simulink model "sampleModel16"  (Simulink 9.1)
settings: Solver=VariableStepAuto  StartTime=0.0  StopTime=10.0  RelTol=1e-3
undefined symbols (not defined in the file): DiscIntNeverNeededParam, Newton, Raphson
libraries: simulink x14
settings Model: SuppressorTable="22 serialization::archive 11 0 6 0 0 1 8 0 0 0 0 6 0 0 1 0 21 sampleModel16/cfblk29 0 6 0 0 2 8 0 0 0 0 6 41 Simulink:DataType:WarningOverFlowDetected 0 0 0 6 0  0  0 0 0 0 8 20160608 0 0 0 15 23 17 0 1 40 SimulinkFixedPoint:util:Overflowoccurred 0 0 0  0  8 20160608 0 15 23 17 0 1"  Creator=DELL  LastModifiedBy=DELL
settings DataIOCC: SaveFormat=Dataset
settings OptimizationCC: LifeSpan=auto
settings DebuggingCC: UnderspecifiedInitializationDetection=Simplified  MergeDetectMultiDrivingBlocksExec=error  SFUnexpectedBacktrackingDiag=error  SFNoUnconditionalDefaultTransitionDiag=error  SFExecutionAtInitializationDiag=warning
settings HardwareCC: ProdBitPerPointer=64  ProdBitPerSizeT=64  ProdBitPerPtrDiffT=64  ProdLargestAtomicFloat=Float  ProdIntDivRoundTo=Zero  ProdEndianess=LittleEndian  ProdWordSize=64  ProdHWDeviceType=Intel->x86-64 (Windows64)
settings ModelReferenceCC: PropagateSignalLabelsOutOfModel=on
settings CodeAppCC: StateflowObjectComments=off
settings GRTTargetCC: TargetLangStandard=C99 (ISO)  CombineOutputUpdateFcns=on  GRTInterface=off
settings ConfigComp: CovMetricSettings=dwe  CovHtmlReporting=off  CovSaveCumulativeToWorkspaceVar=off  CovSaveSingleToWorkspaceVar=off  CovExternalEMLEnable=on

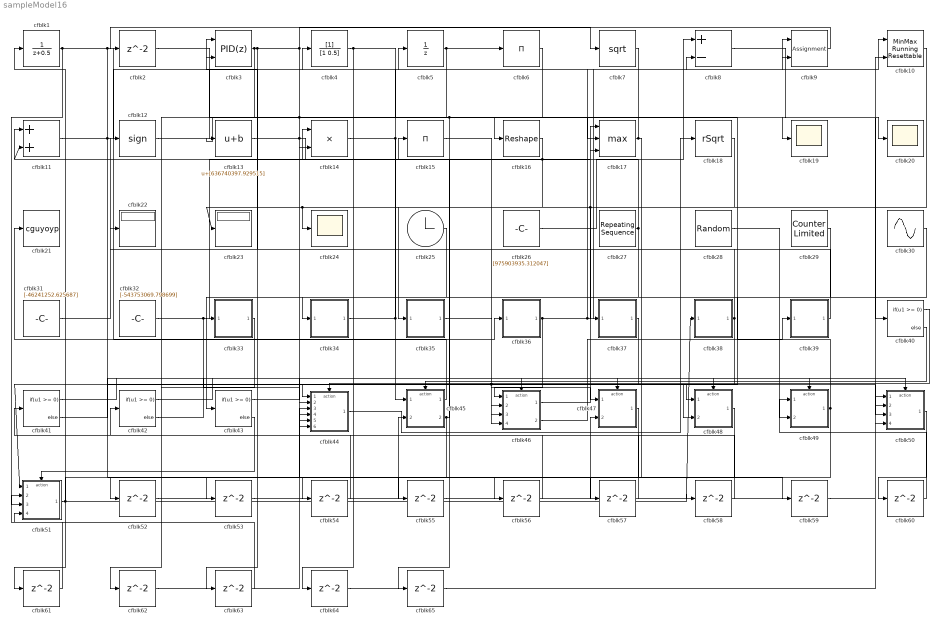
== system sampleModel16 ==
  cfblk1 : DiscreteTransferFcn  SampleTime=1
  cfblk10 : simulink/Math Operations/MinMax Running Resettable  Function=min  vinit=0.0
  cfblk11 : Sum
  cfblk12 : Signum
  cfblk13 : Bias  Bias=[636740397.929515]
  cfblk14 : Product  Inputs=**
  cfblk15 : Product  Inputs=*
  cfblk16 : Reshape
  cfblk17 : MinMax  Function=max  Inputs=3
  cfblk18 : Sqrt  Operator=rSqrt  AlgorithmType=Newton-Raphson  SaturateOnIntegerOverflow=on
  cfblk19 : Scope
  cfblk{2,52..65} (15 alike) : Delay  SampleTime=1
  cfblk20 : Scope
  cfblk21 : ToWorkspace  VariableName=cguyoyp  SaveFormat=Timeseries  SampleTime=-1
  cfblk22 : Display
  cfblk23 : Display
  cfblk24 : Scope
  cfblk25 : Clock
  cfblk26 : Constant  Value=[975903935.312047]  SampleTime=1
  cfblk27 : simulink/Sources/Repeating Sequence  rep_seq_t=[0 2]  rep_seq_y=[-628768262.786288, 33540011.241070]
  cfblk28 : UniformRandomNumber  Minimum=[-3598479047.893037]  Maximum=[8689509005.201536]  Seed=[60011837.000000]  SampleTime=0.1
  cfblk29 : simulink/Sources/Counter Limited  uplimit=[999.000000]  tsamp=-1
  cfblk3 : simulink/Continuous/PID Controller (2DOF)  Controller=PID  TimeDomain=Discrete-time  SampleTime=1  IntegratorMethod=Forward Euler  FilterMethod=Forward Euler  Form=Parallel  UseFilter=on  ControllerParametersSource=internal  P=1  I=1  D=0  N=100  b=1  c=1  InitialConditionSource=internal  InitialConditionForIntegrator=0  InitialConditionForFilter=0  ExternalReset=none  LimitOutput=off  UpperSaturationLimit=inf  LowerSaturationLimit=-inf  LinearizeAsGain=off  AntiWindupMode=none  Kb=1  TrackingMode=off  Kt=1  PParamMin=[]  PParamMax=[]  IParamMin=[]  IParamMax=[]  DParamMin=[]  DParamMax=[]  NParamMin=[]  NParamMax=[]  bParamMin=[]  bParamMax=[]  cParamMin=[]  cParamMax=[]  KbParamMin=[]  KbParamMax=[]  KtParamMin=[]  KtParamMax=[]  POutMin=[]  POutMax=[]  IOutMin=[]  IOutMax=[]  DOutMin=[]  DOutMax=[]  NOutMin=[]  NOutMax=[]  bOutMin=[]  bOutMax=[]  cOutMin=[]  cOutMax=[]  KbOutMin=[]  KbOutMax=[]  KtOutMin=[]  KtOutMax=[]  IntegratorOutMin=[]  IntegratorOutMax=[]  FilterOutMin=[]  FilterOutMax=[]  SumOutMin=[]  SumOutMax=[]  Sum1OutMin=[]  Sum1OutMax=[]  Sum2OutMin=[]  Sum2OutMax=[]  Sum3OutMin=[]  Sum3OutMax=[]  SumI1OutMin=[]  SumI1OutMax=[]  SumI2OutMin=[]  SumI2OutMax=[]  SumI3OutMin=[]  SumI3OutMax=[]  SumDOutMin=[]  SumDOutMax=[]  SaturationOutMin=[]  SaturationOutMax=[]  IntegratorContinuousStateAttributes=''  IntegratorStateMustResolveToSignalObject=off  IntegratorRTWStateStorageClass=Auto  FilterContinuousStateAttributes=''  FilterStateMustResolveToSignalObject=off  FilterRTWStateStorageClass=Auto  DifferentiatorICPrevScaledInput=0  DifferentiatorOutMin=[]  DifferentiatorOutMax=[]  FilterDiffOutCoefMin=[]  FilterDiffOutCoefMax=[]  SumDenOutMin=[]  SumDenOutMax=[]  SumNumOutMin=[]  SumNumOutMax=[]  ReciprocalOutMin=[]  ReciprocalOutMax=[]  DivideOutMin=[]  DivideOutMax=[]  TunerSelectOption=Transfer Function Based (PID Tuner App)
  cfblk30 : Sin  Amplitude=[-741647399.193095]  Bias=[-413258711.550195]  SampleTime=0
  cfblk31 : Constant  Value=[-46241252.625687]  SampleTime=1
  cfblk32 : Constant  Value=[-543753069.798699]  SampleTime=1
  cfblk33 : Subsystem
  cfblk34 : Subsystem
  cfblk35 : Subsystem
  cfblk36 : Subsystem
  cfblk37 : Subsystem
  cfblk38 : Subsystem
  cfblk39 : Subsystem
  cfblk4 : DiscreteFilter  SampleTime=1
  cfblk{40..43} (4 alike) : If  IfExpression=u1 >= 0  SampleTime=1
  cfblk44 : Subsystem  TreatAsAtomicUnit=on
  cfblk45 : Subsystem  TreatAsAtomicUnit=on
  cfblk46 : Subsystem  TreatAsAtomicUnit=on
  cfblk47 : Subsystem  TreatAsAtomicUnit=on
  cfblk48 : Subsystem  TreatAsAtomicUnit=on
  cfblk49 : Subsystem  TreatAsAtomicUnit=on
  cfblk5 : UnitDelay
  cfblk50 : Subsystem  TreatAsAtomicUnit=on
  cfblk51 : Subsystem  TreatAsAtomicUnit=on
  cfblk6 : Product  Inputs=*
  cfblk7 : Sqrt  SaturateOnIntegerOverflow=on
  cfblk8 : Sum  Inputs=+-
  cfblk9 : Assignment  DiagnosticForDimensions=Warning  IndexOptions=Index vector (dialog)  Indices=1  OutputSizes=1
  wires:
  cfblk12/1 -> cfblk5/1
  cfblk32/1 -> cfblk15/1, cfblk44/6(cfblk17)
  cfblk51/1(cfblk2) -> cfblk38/1(cfblk1), cfblk11/1
  cfblk37/1(cfblk2) -> cfblk51/1(cfblk1), cfblk46/2(cfblk10)
  cfblk49/1(cfblk2) -> cfblk13/1, cfblk61/1
  cfblk8/1 -> cfblk20/1
  cfblk1/1 -> cfblk36/1(cfblk1), cfblk50/3(cfblk15), cfblk51/3(cfblk13)
  cfblk9/1 -> cfblk2/1
  cfblk36/1(cfblk2) -> cfblk10/1, cfblk9/1, cfblk46/1(cfblk1)
  cfblk45/1(cfblk2) -> cfblk21/1
  cfblk44/1(cfblk2) -> cfblk18/1
  cfblk29/1 -> cfblk43/1
  cfblk26/1 -> cfblk8/1
  cfblk16/1 -> cfblk23/1, cfblk24/1, cfblk11/2
  cfblk11/1 -> cfblk4/1, cfblk55/1
  cfblk17/1 -> cfblk16/1, cfblk57/1
  cfblk14/1 -> cfblk8/2, cfblk46/3(cfblk11)
  cfblk45/2(cfblk12) -> cfblk14/1, cfblk64/1
  cfblk46/1(cfblk2) -> cfblk17/1
  cfblk38/1(cfblk2) -> cfblk12/1, cfblk44/1(cfblk1)
  cfblk2/1 -> cfblk40/1
  cfblk3/1 -> cfblk7/1, cfblk58/1, cfblk63/1, cfblk62/1
  cfblk31/1 -> cfblk22/1
  cfblk10/1 -> cfblk37/1(cfblk1), cfblk46/4(cfblk12)
  cfblk15/1 -> cfblk47/1(cfblk1)
  cfblk13/1 -> cfblk17/3, cfblk59/1
  cfblk25/1 -> cfblk34/1(cfblk1)
  cfblk5/1 -> cfblk6/1, cfblk14/2
  cfblk27/1 -> cfblk3/1, cfblk44/2(cfblk13)
  cfblk30/1 -> cfblk48/1(cfblk1)
  cfblk7/1 -> cfblk17/2
  cfblk18/1 -> cfblk35/1(cfblk1)
  cfblk28/1 -> cfblk49/2(cfblk17)
  cfblk35/1(cfblk2) -> cfblk48/2(cfblk10)
  cfblk34/1(cfblk2) -> cfblk45/1(cfblk1), cfblk9/2
  cfblk4/1 -> cfblk19/1, cfblk54/1
  cfblk6/1 -> cfblk33/1(cfblk1), cfblk44/4(cfblk15), cfblk65/1
  cfblk46/2(cfblk13) -> cfblk39/1(cfblk1)
  cfblk39/1(cfblk2) -> cfblk3/2
  cfblk40/1 -> cfblk44/Action
  cfblk40/2 -> cfblk45/Action
  cfblk41/1 -> cfblk46/Action
  cfblk41/2 -> cfblk47/Action
  cfblk42/1 -> cfblk48/Action
  cfblk42/2 -> cfblk49/Action
  cfblk43/1 -> cfblk50/Action
  cfblk43/2 -> cfblk51/Action
  cfblk33/1(cfblk2) -> cfblk52/1
  cfblk52/1 -> cfblk10/2
  cfblk48/1(cfblk2) -> cfblk53/1
  cfblk53/1 -> cfblk45/2(cfblk11)
  cfblk54/1 -> cfblk1/1
  cfblk55/1 -> cfblk47/2(cfblk10)
  cfblk47/1(cfblk2) -> cfblk56/1
  cfblk56/1 -> cfblk41/1
  cfblk57/1 -> cfblk44/5(cfblk16)
  cfblk58/1 -> cfblk42/1
  cfblk59/1 -> cfblk50/1(cfblk1)
  cfblk50/1(cfblk2) -> cfblk60/1
  cfblk60/1 -> cfblk49/1(cfblk1)
  cfblk61/1 -> cfblk51/2(cfblk12)
  cfblk62/1 -> cfblk44/3(cfblk14)
  cfblk63/1 -> cfblk51/4(cfblk14)
  cfblk64/1 -> cfblk50/2(cfblk14)
  cfblk65/1 -> cfblk50/4(cfblk16)

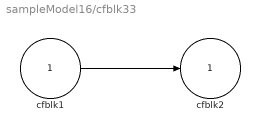
== system sampleModel16/cfblk33 ==
  cfblk1 : Inport
  cfblk2 : Outport
  wires:
  cfblk1/1 -> cfblk2/1

== system sampleModel16/cfblk34 ==
  cfblk1 : Inport
  cfblk2 : Outport
  wires:
  cfblk1/1 -> cfblk2/1

== system sampleModel16/cfblk35 ==
  cfblk1 : Inport
  cfblk2 : Outport
  wires:
  cfblk1/1 -> cfblk2/1

== system sampleModel16/cfblk36 ==
  cfblk1 : Inport
  cfblk2 : Outport
  wires:
  cfblk1/1 -> cfblk2/1

== system sampleModel16/cfblk37 ==
  cfblk1 : Inport
  cfblk2 : Outport
  wires:
  cfblk1/1 -> cfblk2/1

== system sampleModel16/cfblk38 ==
  cfblk1 : Inport
  cfblk2 : Outport
  wires:
  cfblk1/1 -> cfblk2/1

== system sampleModel16/cfblk39 ==
  cfblk1 : Inport
  cfblk2 : Outport
  wires:
  cfblk1/1 -> cfblk2/1

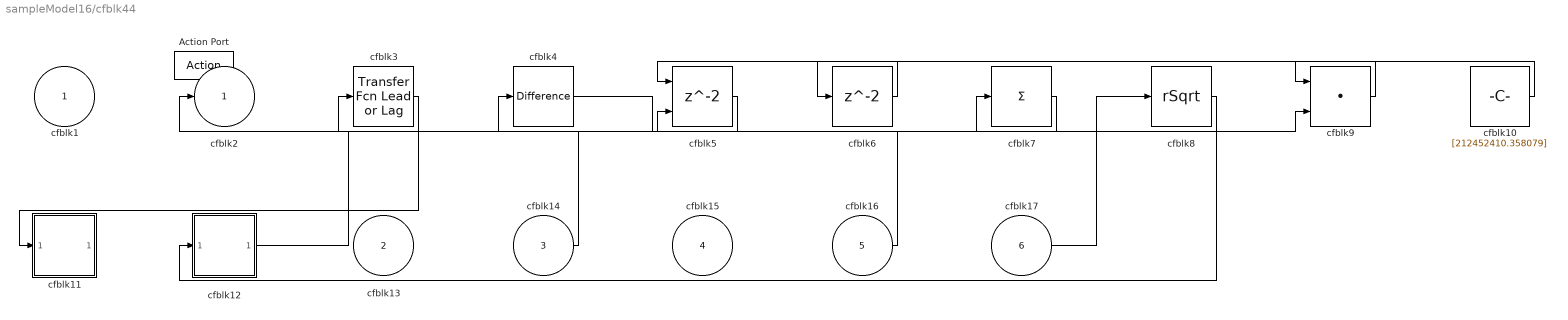
== system sampleModel16/cfblk44 ==
  cfblk1 : Inport
  cfblk13 : Inport  Port=2
  cfblk14 : Inport  Port=3
  cfblk15 : Inport  Port=4
  cfblk16 : Inport  Port=5
  cfblk17 : Inport  Port=6
  Action Port : ActionPort  ActionType=then
  cfblk10 : Constant  Value=[212452410.358079]  SampleTime=1
  cfblk11 : Subsystem
  cfblk12 : Subsystem
  cfblk3 : simulink/Discrete/Transfer Fcn Lead or Lag  PoleZ=0.95  ZeroZ=0.75  ICPrevOutput=0.0  ICPrevInput=0.0  DoSatur=off
      settings: SourceProductName=Simulink  SourceProductBaseCode=SL
  cfblk4 : simulink/Discrete/Difference  ICPrevInput=0.0  OutMin=[]  OutMax=[]  OutDataTypeStr=Inherit: Inherit via back propagation  OutDataType=fixdt(1, 16)  OutScaling=2^-10  DoSatur=off
  cfblk5 : Delay  ShowEnablePort=on
      settings: InputPortMap=u0,e6
  cfblk6 : Delay
  cfblk7 : Sum  Inputs=+
  cfblk8 : Sqrt  Operator=rSqrt  AlgorithmType=Newton-Raphson  SaturateOnIntegerOverflow=on
  cfblk9 : DotProduct  InputSameDT=on  OutDataTypeStr=Inherit: Inherit via internal rule
  cfblk2 : Outport
  wires:
  cfblk3/1 -> cfblk11/1(cfblk1)
  cfblk6/1 -> cfblk5/1
  cfblk14/1 -> cfblk4/1
  cfblk7/1 -> cfblk5/2
  cfblk5/1 -> cfblk2/1
  cfblk10/1 -> cfblk9/1
  cfblk17/1 -> cfblk8/1
  cfblk12/1(cfblk2) -> cfblk7/1
  cfblk8/1 -> cfblk12/1(cfblk1)
  cfblk9/1 -> cfblk6/1
  cfblk4/1 -> cfblk9/2
  cfblk16/1 -> cfblk3/1

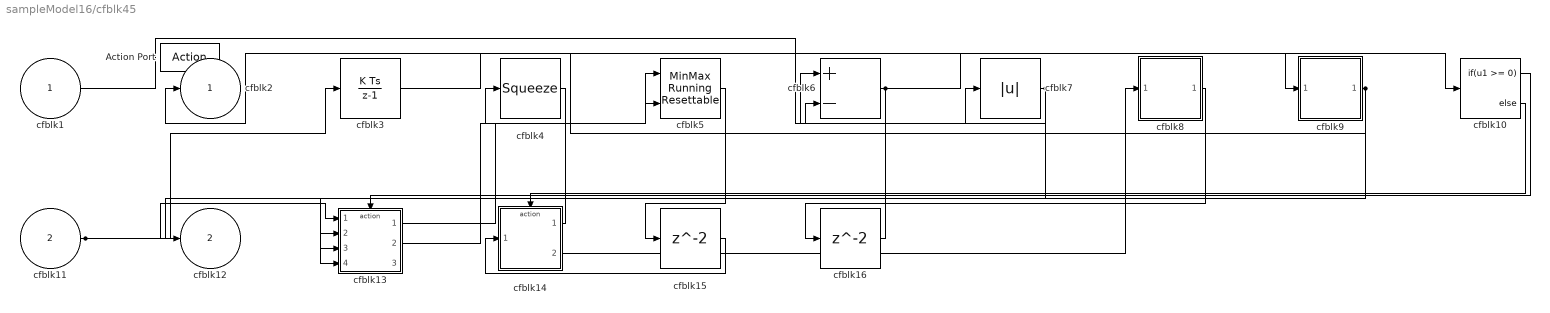
== system sampleModel16/cfblk45 ==
  cfblk1 : Inport
  cfblk11 : Inport  Port=2
  Action Port : ActionPort  ActionType=else
  cfblk10 : If  IfExpression=u1 >= 0  SampleTime=1
  cfblk13 : Subsystem  TreatAsAtomicUnit=on
  cfblk14 : Subsystem  TreatAsAtomicUnit=on
  cfblk15 : Delay
  cfblk16 : Delay
  cfblk3 : DiscreteIntegrator  SampleTime=-1  ICPrevOutput=DiscIntNeverNeededParam  ICPrevScaledInput=DiscIntNeverNeededParam
  cfblk4 : Squeeze
  cfblk5 : simulink/Math Operations/MinMax Running Resettable  Function=min  vinit=0.0
  cfblk6 : Sum  Inputs=+-
  cfblk7 : Abs
  cfblk8 : Subsystem
  cfblk9 : Subsystem
  cfblk2 : Outport
  cfblk12 : Outport  Port=2
  wires:
  cfblk14/1(cfblk2) -> cfblk4/1
  cfblk1/1 -> cfblk7/1
  cfblk9/1(cfblk2) -> cfblk2/1, cfblk13/3(cfblk12)
  cfblk6/1 -> cfblk10/1, cfblk13/2(cfblk11)
  cfblk11/1 -> cfblk3/1, cfblk13/1(cfblk1)
  cfblk14/2(cfblk16) -> cfblk8/1(cfblk1)
  cfblk7/1 -> cfblk6/2, cfblk13/4(cfblk13)
  cfblk4/1 -> cfblk12/1
  cfblk3/1 -> cfblk9/1(cfblk1)
  cfblk13/1(cfblk2) -> cfblk5/1
  cfblk13/2(cfblk14) -> cfblk5/2
  cfblk10/1 -> cfblk13/Action
  cfblk10/2 -> cfblk14/Action
  cfblk5/1 -> cfblk15/1
  cfblk15/1 -> cfblk14/1(cfblk1)
  cfblk8/1(cfblk2) -> cfblk16/1
  cfblk16/1 -> cfblk6/1

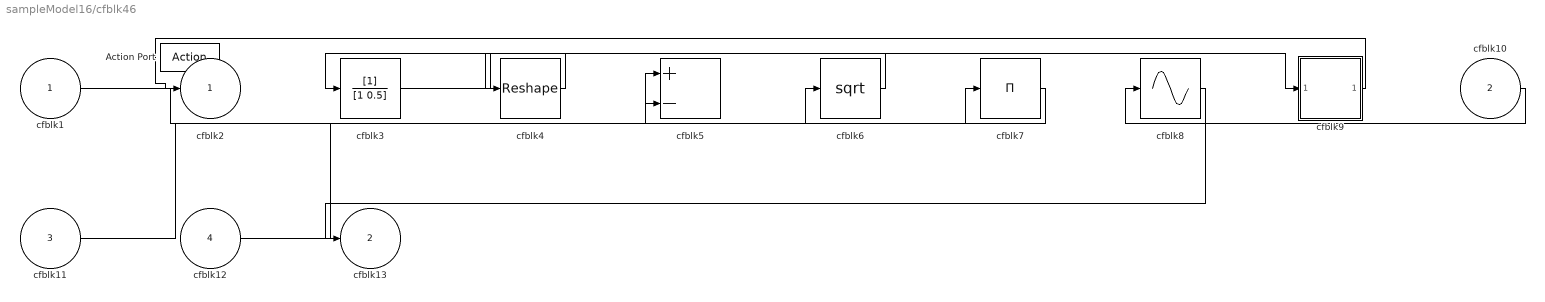
== system sampleModel16/cfblk46 ==
  cfblk1 : Inport
  cfblk10 : Inport  Port=2
  cfblk11 : Inport  Port=3
  cfblk12 : Inport  Port=4
  Action Port : ActionPort  ActionType=then
  cfblk3 : DiscreteFilter
  cfblk4 : Reshape
  cfblk5 : Sum  Inputs=+-
  cfblk6 : Sqrt  SaturateOnIntegerOverflow=on
  cfblk7 : Product  Inputs=*
  cfblk8 : Sin  TimeSource=Use external signal  SampleTime=0
  cfblk9 : Subsystem
  cfblk2 : Outport
  cfblk13 : Outport  Port=2
  wires:
  cfblk12/1 -> cfblk6/1
  cfblk3/1 -> cfblk9/1(cfblk1)
  cfblk4/1 -> cfblk3/1
  cfblk1/1 -> cfblk7/1
  cfblk11/1 -> cfblk5/1
  cfblk10/1 -> cfblk8/1
  cfblk6/1 -> cfblk4/1
  cfblk9/1(cfblk2) -> cfblk2/1
  cfblk8/1 -> cfblk13/1
  cfblk7/1 -> cfblk5/2

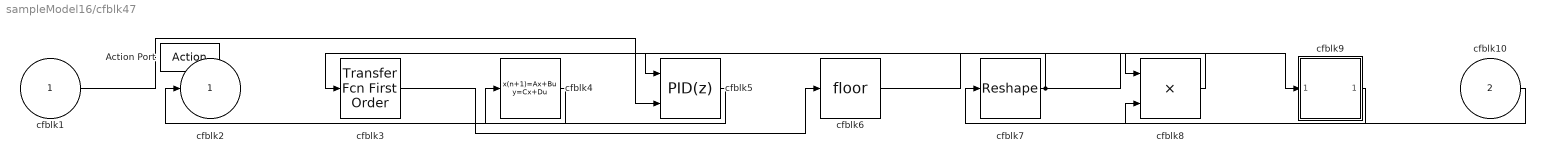
== system sampleModel16/cfblk47 ==
  cfblk1 : Inport
  cfblk10 : Inport  Port=2
  Action Port : ActionPort  ActionType=else
  cfblk3 : simulink/Discrete/Transfer Fcn First Order  PoleZ=0.95  ICPrevOutput=0.0  DoSatur=off
      settings: SourceProductName=Simulink
  cfblk4 : DiscreteStateSpace  SampleTime=-1
  cfblk5 : simulink/Continuous/PID Controller (2DOF)  Controller=PID  TimeDomain=Discrete-time  SampleTime=-1  IntegratorMethod=Forward Euler  FilterMethod=Forward Euler  Form=Parallel  UseFilter=on  ControllerParametersSource=internal  P=1  I=1  D=0  N=100  b=1  c=1  InitialConditionSource=internal  InitialConditionForIntegrator=0  InitialConditionForFilter=0  ExternalReset=none  LimitOutput=off  UpperSaturationLimit=inf  LowerSaturationLimit=-inf  LinearizeAsGain=off  AntiWindupMode=none  Kb=1  TrackingMode=off  Kt=1  PParamMin=[]  PParamMax=[]  IParamMin=[]  IParamMax=[]  DParamMin=[]  DParamMax=[]  NParamMin=[]  NParamMax=[]  bParamMin=[]  bParamMax=[]  cParamMin=[]  cParamMax=[]  KbParamMin=[]  KbParamMax=[]  KtParamMin=[]  KtParamMax=[]  POutMin=[]  POutMax=[]  IOutMin=[]  IOutMax=[]  DOutMin=[]  DOutMax=[]  NOutMin=[]  NOutMax=[]  bOutMin=[]  bOutMax=[]  cOutMin=[]  cOutMax=[]  KbOutMin=[]  KbOutMax=[]  KtOutMin=[]  KtOutMax=[]  IntegratorOutMin=[]  IntegratorOutMax=[]  FilterOutMin=[]  FilterOutMax=[]  SumOutMin=[]  SumOutMax=[]  Sum1OutMin=[]  Sum1OutMax=[]  Sum2OutMin=[]  Sum2OutMax=[]  Sum3OutMin=[]  Sum3OutMax=[]  SumI1OutMin=[]  SumI1OutMax=[]  SumI2OutMin=[]  SumI2OutMax=[]  SumI3OutMin=[]  SumI3OutMax=[]  SumDOutMin=[]  SumDOutMax=[]  SaturationOutMin=[]  SaturationOutMax=[]  IntegratorContinuousStateAttributes=''  IntegratorStateMustResolveToSignalObject=off  IntegratorRTWStateStorageClass=Auto  FilterContinuousStateAttributes=''  FilterStateMustResolveToSignalObject=off  FilterRTWStateStorageClass=Auto  DifferentiatorICPrevScaledInput=0  DifferentiatorOutMin=[]  DifferentiatorOutMax=[]  FilterDiffOutCoefMin=[]  FilterDiffOutCoefMax=[]  SumDenOutMin=[]  SumDenOutMax=[]  SumNumOutMin=[]  SumNumOutMax=[]  ReciprocalOutMin=[]  ReciprocalOutMax=[]  DivideOutMin=[]  DivideOutMax=[]  TunerSelectOption=Transfer Function Based (PID Tuner App)
  cfblk6 : Rounding
  cfblk7 : Reshape
  cfblk8 : Product
  cfblk9 : Subsystem
  cfblk2 : Outport
  wires:
  cfblk8/1 -> cfblk5/1
  cfblk10/1 -> cfblk7/1
  cfblk5/1 -> cfblk4/1
  cfblk1/1 -> cfblk5/2
  cfblk6/1 -> cfblk8/1
  cfblk7/1 -> cfblk3/1, cfblk9/1(cfblk1)
  cfblk3/1 -> cfblk6/1
  cfblk4/1 -> cfblk2/1
  cfblk9/1(cfblk2) -> cfblk8/2

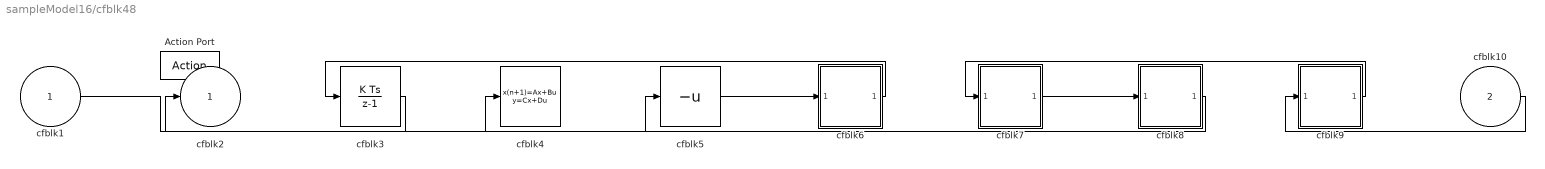
== system sampleModel16/cfblk48 ==
  cfblk1 : Inport
  cfblk10 : Inport  Port=2
  Action Port : ActionPort  ActionType=then
  cfblk3 : DiscreteIntegrator  SampleTime=-1  ICPrevOutput=DiscIntNeverNeededParam  ICPrevScaledInput=DiscIntNeverNeededParam
  cfblk4 : DiscreteStateSpace  SampleTime=-1
  cfblk5 : UnaryMinus
  cfblk6 : Subsystem
  cfblk7 : Subsystem
  cfblk8 : Subsystem
  cfblk9 : Subsystem
  cfblk2 : Outport
  wires:
  cfblk3/1 -> cfblk2/1
  cfblk9/1(cfblk2) -> cfblk7/1(cfblk1)
  cfblk5/1 -> cfblk6/1(cfblk1)
  cfblk8/1(cfblk2) -> cfblk4/1
  cfblk7/1(cfblk2) -> cfblk8/1(cfblk1)
  cfblk6/1(cfblk2) -> cfblk3/1
  cfblk10/1 -> cfblk9/1(cfblk1)
  cfblk1/1 -> cfblk5/1

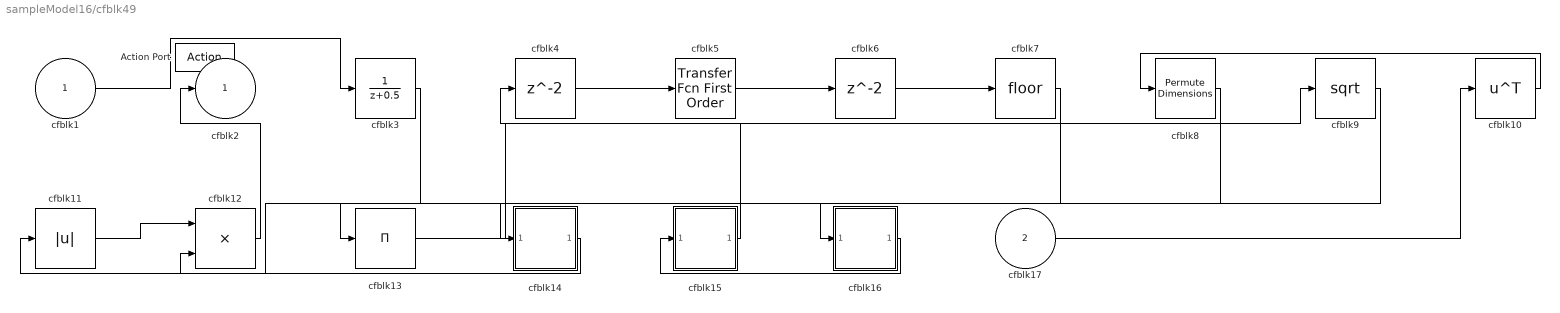
== system sampleModel16/cfblk49 ==
  cfblk1 : Inport
  cfblk17 : Inport  Port=2
  Action Port : ActionPort  ActionType=else
  cfblk10 : Math  Operator=transpose  SaturateOnIntegerOverflow=on
  cfblk11 : Abs
  cfblk12 : Product  Inputs=**
  cfblk13 : Product  Inputs=*
  cfblk14 : Subsystem
  cfblk15 : Subsystem
  cfblk16 : Subsystem
  cfblk3 : DiscreteTransferFcn
  cfblk4 : Delay
  cfblk5 : simulink/Discrete/Transfer Fcn First Order  PoleZ=0.95  ICPrevOutput=0.0  DoSatur=off
      settings: SourceProductName=Simulink
  cfblk6 : Delay
  cfblk7 : Rounding
  cfblk8 : PermuteDimensions
  cfblk9 : Sqrt  SaturateOnIntegerOverflow=on
  cfblk2 : Outport
  wires:
  cfblk4/1 -> cfblk5/1
  cfblk17/1 -> cfblk10/1
  cfblk11/1 -> cfblk12/1
  cfblk5/1 -> cfblk6/1
  cfblk12/1 -> cfblk2/1
  cfblk9/1 -> cfblk11/1
  cfblk16/1(cfblk2) -> cfblk15/1(cfblk1)
  cfblk3/1 -> cfblk13/1
  cfblk14/1(cfblk2) -> cfblk12/2
  cfblk13/1 -> cfblk9/1
  cfblk8/1 -> cfblk16/1(cfblk1)
  cfblk1/1 -> cfblk3/1
  cfblk15/1(cfblk2) -> cfblk4/1
  cfblk10/1 -> cfblk8/1
  cfblk6/1 -> cfblk7/1
  cfblk7/1 -> cfblk14/1(cfblk1)

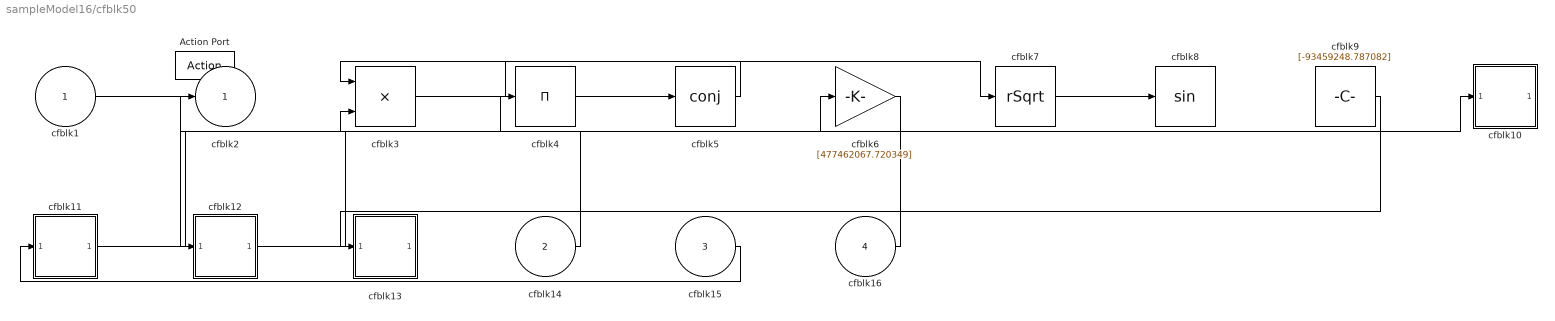
== system sampleModel16/cfblk50 ==
  cfblk1 : Inport
  cfblk14 : Inport  Port=2
  cfblk15 : Inport  Port=3
  cfblk16 : Inport  Port=4
  Action Port : ActionPort  ActionType=then
  cfblk10 : Subsystem
  cfblk11 : Subsystem
  cfblk12 : Subsystem
  cfblk13 : Subsystem
  cfblk3 : Product
  cfblk4 : Product  Inputs=*
  cfblk5 : Math  Operator=conj  SaturateOnIntegerOverflow=on
  cfblk6 : Gain  Gain=[477462067.720349]
  cfblk7 : Sqrt  Operator=rSqrt  AlgorithmType=Newton-Raphson  SaturateOnIntegerOverflow=on
  cfblk8 : Trigonometry
  cfblk9 : Constant  Value=[-93459248.787082]  SampleTime=1
  cfblk2 : Outport
  wires:
  cfblk11/1(cfblk2) -> cfblk10/1(cfblk1)
  cfblk15/1 -> cfblk11/1(cfblk1)
  cfblk3/1 -> cfblk7/1
  cfblk7/1 -> cfblk8/1
  cfblk12/1(cfblk2) -> cfblk6/1
  cfblk1/1 -> cfblk12/1(cfblk1)
  cfblk5/1 -> cfblk3/1
  cfblk9/1 -> cfblk13/1(cfblk1)
  cfblk14/1 -> cfblk4/1
  cfblk6/1 -> cfblk2/1
  cfblk16/1 -> cfblk3/2
  cfblk4/1 -> cfblk5/1

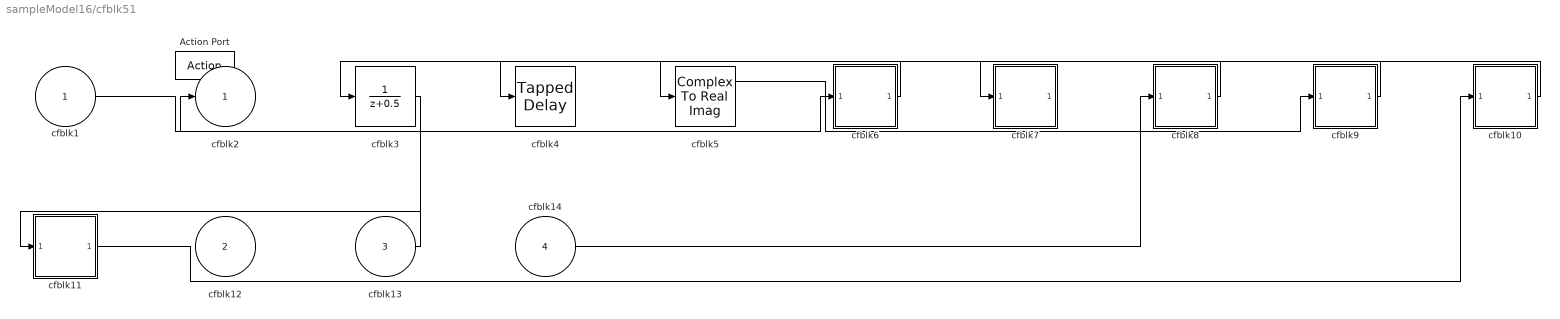
== system sampleModel16/cfblk51 ==
  cfblk1 : Inport
  cfblk12 : Inport  Port=2
  cfblk13 : Inport  Port=3
  cfblk14 : Inport  Port=4
  Action Port : ActionPort  ActionType=else
  cfblk10 : Subsystem
  cfblk11 : Subsystem
  cfblk3 : DiscreteTransferFcn
  cfblk4 : simulink/Discrete/Tapped Delay  vinit=0.0  samptime=-1  NumDelays=1  DelayOrder=Oldest  includeCurrent=off
  cfblk5 : ComplexToRealImag
  cfblk6 : Subsystem
  cfblk7 : Subsystem
  cfblk8 : Subsystem
  cfblk9 : Subsystem
  cfblk2 : Outport
  wires:
  cfblk9/1(cfblk2) -> cfblk7/1(cfblk1)
  cfblk13/1 -> cfblk2/1
  cfblk11/1(cfblk2) -> cfblk10/1(cfblk1)
  cfblk5/1 -> cfblk9/1(cfblk1)
  cfblk6/1(cfblk2) -> cfblk3/1
  cfblk14/1 -> cfblk8/1(cfblk1)
  cfblk10/1(cfblk2) -> cfblk4/1
  cfblk8/1(cfblk2) -> cfblk5/1
  cfblk1/1 -> cfblk6/1(cfblk1)
  cfblk3/1 -> cfblk11/1(cfblk1)

== system sampleModel16/cfblk44/cfblk11 ==
  cfblk1 : Inport
  cfblk2 : Outport
  wires:
  cfblk1/1 -> cfblk2/1

== system sampleModel16/cfblk44/cfblk12 ==
  cfblk1 : Inport
  cfblk2 : Outport
  wires:
  cfblk1/1 -> cfblk2/1

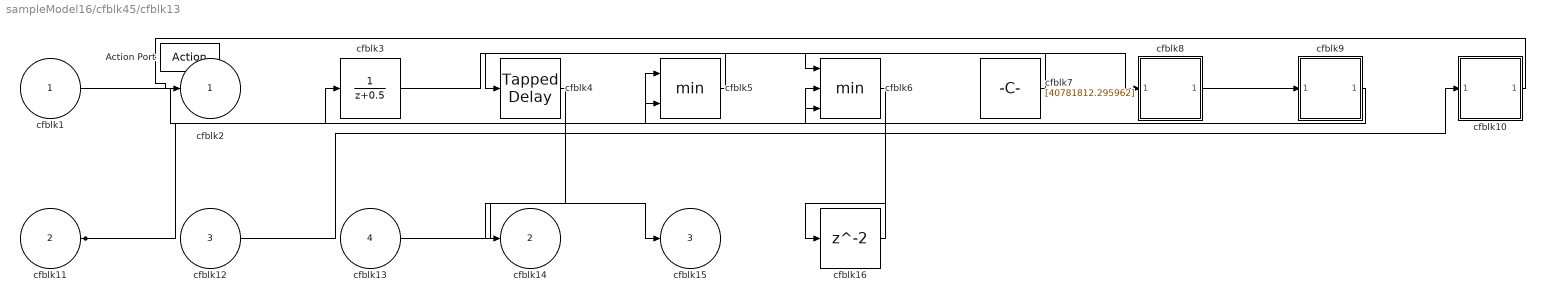
== system sampleModel16/cfblk45/cfblk13 ==
  cfblk1 : Inport
  cfblk11 : Inport  Port=2
  cfblk12 : Inport  Port=3
  cfblk13 : Inport  Port=4
  Action Port : ActionPort  ActionType=then
  cfblk10 : Subsystem
  cfblk16 : Delay
  cfblk3 : DiscreteTransferFcn
  cfblk4 : simulink/Discrete/Tapped Delay  vinit=0.0  samptime=-1  NumDelays=1  DelayOrder=Oldest  includeCurrent=off
  cfblk5 : MinMax  Inputs=2
  cfblk6 : MinMax  Inputs=3
  cfblk7 : Constant  Value=[40781812.295962]  SampleTime=1
  cfblk8 : Subsystem
  cfblk9 : Subsystem
  cfblk2 : Outport
  cfblk14 : Outport  Port=2
  cfblk15 : Outport  Port=3
  wires:
  cfblk5/1 -> cfblk4/1
  cfblk11/1 -> cfblk5/1, cfblk6/3
  cfblk12/1 -> cfblk10/1(cfblk1)
  cfblk8/1(cfblk2) -> cfblk9/1(cfblk1)
  cfblk7/1 -> cfblk6/1
  cfblk13/1 -> cfblk15/1
  cfblk1/1 -> cfblk5/2
  cfblk9/1(cfblk2) -> cfblk6/2
  cfblk10/1(cfblk2) -> cfblk2/1
  cfblk4/1 -> cfblk14/1
  cfblk3/1 -> cfblk8/1(cfblk1)
  cfblk6/1 -> cfblk16/1
  cfblk16/1 -> cfblk3/1

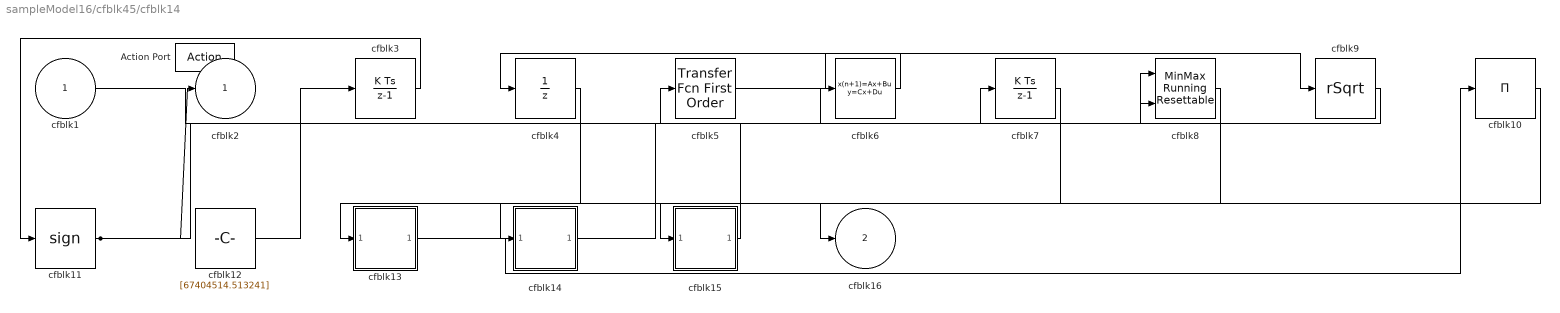
== system sampleModel16/cfblk45/cfblk14 ==
  cfblk1 : Inport
  Action Port : ActionPort  ActionType=else
  cfblk10 : Product  Inputs=*
  cfblk11 : Signum
  cfblk12 : Constant  Value=[67404514.513241]  SampleTime=1
  cfblk13 : Subsystem
  cfblk14 : Subsystem
  cfblk15 : Subsystem
  cfblk3 : DiscreteIntegrator  SampleTime=-1  ICPrevOutput=DiscIntNeverNeededParam  ICPrevScaledInput=DiscIntNeverNeededParam
  cfblk4 : UnitDelay  SampleTime=-1
  cfblk5 : simulink/Discrete/Transfer Fcn First Order  PoleZ=0.95  ICPrevOutput=0.0  DoSatur=off
      settings: SourceProductName=Simulink
  cfblk6 : DiscreteStateSpace  SampleTime=-1
  cfblk7 : DiscreteIntegrator  SampleTime=-1  ICPrevOutput=DiscIntNeverNeededParam  ICPrevScaledInput=DiscIntNeverNeededParam
  cfblk8 : simulink/Math Operations/MinMax Running Resettable  Function=min  vinit=0.0
  cfblk9 : Sqrt  Operator=rSqrt  AlgorithmType=Newton-Raphson  SaturateOnIntegerOverflow=on
  cfblk2 : Outport
  cfblk16 : Outport  Port=2
  wires:
  cfblk5/1 -> cfblk9/1
  cfblk12/1 -> cfblk3/1
  cfblk9/1 -> cfblk7/1
  cfblk8/1 -> cfblk13/1(cfblk1)
  cfblk13/1(cfblk2) -> cfblk10/1
  cfblk4/1 -> cfblk14/1(cfblk1)
  cfblk10/1 -> cfblk15/1(cfblk1)
  cfblk1/1 -> cfblk8/1
  cfblk3/1 -> cfblk11/1
  cfblk7/1 -> cfblk16/1
  cfblk15/1(cfblk2) -> cfblk5/1
  cfblk11/1 -> cfblk2/1, cfblk6/1
  cfblk14/1(cfblk2) -> cfblk8/2
  cfblk6/1 -> cfblk4/1

== system sampleModel16/cfblk45/cfblk8 ==
  cfblk1 : Inport
  cfblk2 : Outport
  wires:
  cfblk1/1 -> cfblk2/1

== system sampleModel16/cfblk45/cfblk9 ==
  cfblk1 : Inport
  cfblk2 : Outport
  wires:
  cfblk1/1 -> cfblk2/1

== system sampleModel16/cfblk46/cfblk9 ==
  cfblk1 : Inport
  cfblk2 : Outport
  wires:
  cfblk1/1 -> cfblk2/1

== system sampleModel16/cfblk47/cfblk9 ==
  cfblk1 : Inport
  cfblk2 : Outport
  wires:
  cfblk1/1 -> cfblk2/1

== system sampleModel16/cfblk48/cfblk6 ==
  cfblk1 : Inport
  cfblk2 : Outport
  wires:
  cfblk1/1 -> cfblk2/1

== system sampleModel16/cfblk48/cfblk7 ==
  cfblk1 : Inport
  cfblk2 : Outport
  wires:
  cfblk1/1 -> cfblk2/1

== system sampleModel16/cfblk48/cfblk8 ==
  cfblk1 : Inport
  cfblk2 : Outport
  wires:
  cfblk1/1 -> cfblk2/1

== system sampleModel16/cfblk48/cfblk9 ==
  cfblk1 : Inport
  cfblk2 : Outport
  wires:
  cfblk1/1 -> cfblk2/1

== system sampleModel16/cfblk49/cfblk14 ==
  cfblk1 : Inport
  cfblk2 : Outport
  wires:
  cfblk1/1 -> cfblk2/1

== system sampleModel16/cfblk49/cfblk15 ==
  cfblk1 : Inport
  cfblk2 : Outport
  wires:
  cfblk1/1 -> cfblk2/1

== system sampleModel16/cfblk49/cfblk16 ==
  cfblk1 : Inport
  cfblk2 : Outport
  wires:
  cfblk1/1 -> cfblk2/1

== system sampleModel16/cfblk50/cfblk10 ==
  cfblk1 : Inport
  cfblk2 : Outport
  wires:
  cfblk1/1 -> cfblk2/1

== system sampleModel16/cfblk50/cfblk11 ==
  cfblk1 : Inport
  cfblk2 : Outport
  wires:
  cfblk1/1 -> cfblk2/1

== system sampleModel16/cfblk50/cfblk12 ==
  cfblk1 : Inport
  cfblk2 : Outport
  wires:
  cfblk1/1 -> cfblk2/1

== system sampleModel16/cfblk50/cfblk13 ==
  cfblk1 : Inport
  cfblk2 : Outport
  wires:
  cfblk1/1 -> cfblk2/1

== system sampleModel16/cfblk51/cfblk10 ==
  cfblk1 : Inport
  cfblk2 : Outport
  wires:
  cfblk1/1 -> cfblk2/1

== system sampleModel16/cfblk51/cfblk11 ==
  cfblk1 : Inport
  cfblk2 : Outport
  wires:
  cfblk1/1 -> cfblk2/1

== system sampleModel16/cfblk51/cfblk6 ==
  cfblk1 : Inport
  cfblk2 : Outport
  wires:
  cfblk1/1 -> cfblk2/1

== system sampleModel16/cfblk51/cfblk7 ==
  cfblk1 : Inport
  cfblk2 : Outport
  wires:
  cfblk1/1 -> cfblk2/1

== system sampleModel16/cfblk51/cfblk8 ==
  cfblk1 : Inport
  cfblk2 : Outport
  wires:
  cfblk1/1 -> cfblk2/1

== system sampleModel16/cfblk51/cfblk9 ==
  cfblk1 : Inport
  cfblk2 : Outport
  wires:
  cfblk1/1 -> cfblk2/1

== system sampleModel16/cfblk45/cfblk13/cfblk10 ==
  cfblk1 : Inport
  cfblk2 : Outport
  wires:
  cfblk1/1 -> cfblk2/1

== system sampleModel16/cfblk45/cfblk13/cfblk8 ==
  cfblk1 : Inport
  cfblk2 : Outport
  wires:
  cfblk1/1 -> cfblk2/1

== system sampleModel16/cfblk45/cfblk13/cfblk9 ==
  cfblk1 : Inport
  cfblk2 : Outport
  wires:
  cfblk1/1 -> cfblk2/1

== system sampleModel16/cfblk45/cfblk14/cfblk13 ==
  cfblk1 : Inport
  cfblk2 : Outport
  wires:
  cfblk1/1 -> cfblk2/1

== system sampleModel16/cfblk45/cfblk14/cfblk14 ==
  cfblk1 : Inport
  cfblk2 : Outport
  wires:
  cfblk1/1 -> cfblk2/1

== system sampleModel16/cfblk45/cfblk14/cfblk15 ==
  cfblk1 : Inport
  cfblk2 : Outport
  wires:
  cfblk1/1 -> cfblk2/1
